simulink model "deadbeat_controller_model"  (R2015a)
settings: Solver=ode45  StartTime=0.0  StopTime=10.0  RelTol=1e-3
values from neighbouring files (symbols this model uses):
  T = 0.01    [PID_co.m]    (also in PI_co.m; assignment_digital_control.m; deadbeat_co.m; deadbeat_controller.m)
undefined symbols (not defined in the file or in its folder): A, B, C, D
libraries: cstblocks x2
settings Model: Creator=ayush  LastModifiedBy=ayush

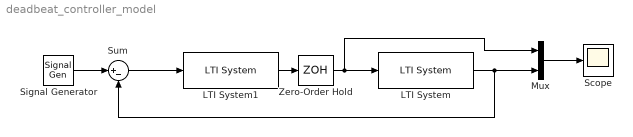
== system deadbeat_controller_model ==
  LTI System : cstblocks/LTI System  sys=ss(A,B,C,D)  IC=[]
  LTI System1 : cstblocks/LTI System  sys=tf(1,[1 1],T)  IC=[]
  Mux : Mux  Inputs=2
  Scope : Scope
  Signal Generator : SignalGenerator  Units=rad/sec
  Sum : Sum  Inputs=|+-
  Zero-Order Hold : ZeroOrderHold  SampleTime=-1
  wires:
  LTI System1/1 -> Zero-Order Hold/1
  LTI System/1 -> Sum/2, Mux/2
  Sum/1 -> LTI System1/1
  Signal Generator/1 -> Sum/1
  Mux/1 -> Scope/1
  Zero-Order Hold/1 -> Mux/1, LTI System/1
